simulink model "test1"  (R2021b)
settings: Solver=VariableStepAuto  StartTime=0.0  StopTime=10.0  RelTol=1e-3
undefined symbols (not defined in the file or in its folder): a, b
settings Model: Creator=is221042  LastModifiedBy=is221042

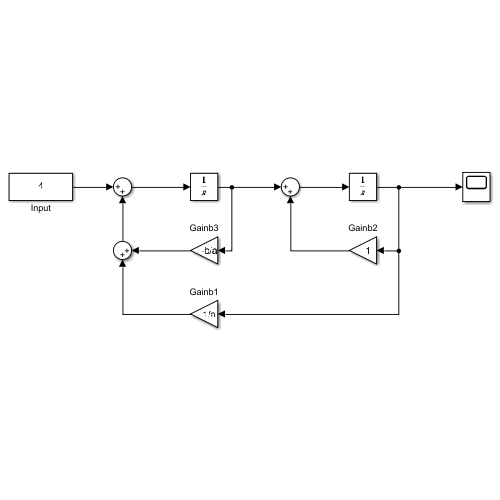
[thumbnail: Simulink's stored preview of the top-level diagram]
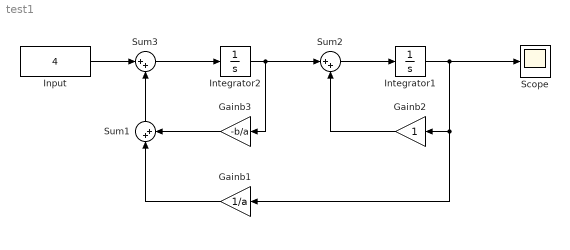
== system test1 ==
  Gainb1 : Gain  Gain=1/a
  Gainb2 : Gain
  Gainb3 : Gain  Gain=-b/a
  Input : Constant  Value=4
  Integrator1 : Integrator
  Integrator2 : Integrator
  Scope : Scope
  Sum1 : Sum  Inputs=|++
  Sum2 : Sum  Inputs=|++
  Sum3 : Sum  Inputs=|++
  wires:
  Integrator2/1 -> Sum2/1, Gainb3/1
  Sum3/1 -> Integrator2/1
  Input/1 -> Sum3/1
  Sum1/1 -> Sum3/2
  Gainb3/1 -> Sum1/2
  Gainb1/1 -> Sum1/1
  Integrator1/1 -> Scope/1, Gainb2/1, Gainb1/1
  Sum2/1 -> Integrator1/1
  Gainb2/1 -> Sum2/2
